simulink model "AdaptiveControlBuilding"  (R2017a)
settings: Solver=FixedStepAuto  StartTime=0  StopTime=75  MaxStep=0.5*Ts  RelTol=1e-3
values from neighbouring files (symbols this model uses):
  Ts = 1    [AdaptiveInitBuilding.m]    (also in Successive_Linearizer_Building.m = 0.5)
  u0 = [op_report.Inputs(1).u;op_report.Inputs(2).u]    [AdaptiveInitBuilding.m]
undefined symbols (not defined in the file or in its folder): K1, K10, K11, K12, K13, K14, K15, K2, K3, K4, K5, K6, K7, K8, K9
libraries: mpclib x1
settings Model: Creator=The MathWorks, Inc.  LastModifiedBy=gaobo1
settings DataIOCC: ExternalInput=ExtIn  InitialState=[311.267; 8.5695]  SaveFormat=Structure  SaveOutput=off  SignalLogging=off  SaveTime=off  SignalLoggingName=logsOut
settings OptimizationCC: BooleanDataType=off  DefaultParameterBehavior=Inlined  InlineInvariantSignals=on  BufferReuse=off  ExpressionDepthLimit=2147483647  InitFltsAndDblsToZero=on  LifeSpan=inf
settings DebuggingCC: SaveWithParameterizedLinksMsg=none  UnderspecifiedInitializationDetection=Classic  MergeDetectMultiDrivingBlocksExec=none  CheckExecutionContextPreStartOutputMsg=on  CheckExecutionContextRuntimeOutputMsg=on  SignalResolutionControl=TryResolveAllWithWarning  MultiTaskDSMMsg=warning  MultiTaskCondExecSysMsg=none  StateNameClashWarn=warning  SFUnexpectedBacktrackingDiag=warning  SFNoUnconditionalDefaultTransitionDiag=warning  SFExecutionAtInitializationDiag=none
settings HardwareCC: ProdBitPerPointer=32  ProdBitPerSizeT=32  ProdBitPerPtrDiffT=32  ProdLargestAtomicFloat=None  ProdIntDivRoundTo=Undefined  ProdEndianess=Unspecified  ProdWordSize=32  ProdHWDeviceType=32-bit Generic  TargetBitPerLong=64  TargetBitPerPointer=64  TargetBitPerSizeT=64  TargetBitPerPtrDiffT=64  TargetLongLongMode=on  TargetIntDivRoundTo=Zero  TargetEndianess=LittleEndian  TargetWordSize=64  TargetHWDeviceType=MATLAB Host  ProdEqTarget=off
settings ModelReferenceCC: PropagateSignalLabelsOutOfModel=off
settings GRTTargetCC: TargetFcnLib=ansi_tfl_tmw.mat  TargetLangStandard=C89/C90 (ANSI)  GeneratePreprocessorConditionals=Disable all  CombineOutputUpdateFcns=off  GRTInterface=on
settings ConfigComp: CovMetricSettings=dw  CovHtmlReporting=on  CovSaveCumulativeToWorkspaceVar=on  CovSaveSingleToWorkspaceVar=on  CovExternalEMLEnable=off  CovSFcnEnable=off

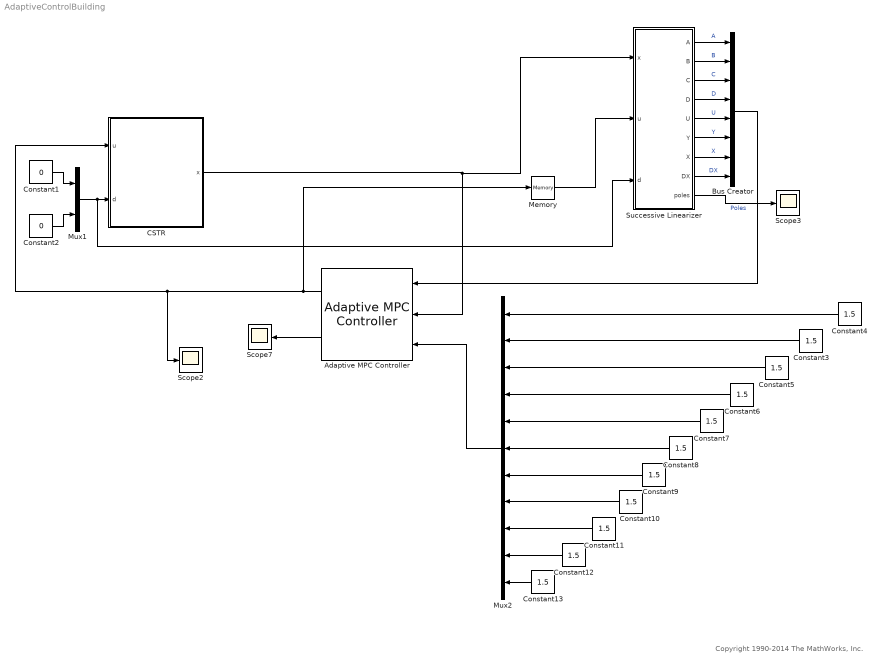
== system AdaptiveControlBuilding ==
  note: Copyright 1990-2014 The MathWorks, Inc.
  Adaptive MPC Controller : mpclib/Adaptive MPC Controller  SCDEnableBlockLinearizationSpecification=on  mpcobj=mpcobj  md_inport=off  mv_inport=off  cost_outport=off  return_sequence=off  return_qpstatus=off  return_state=on  state_inport=off  isltv_plant=off  lims_inport=off  ywt_inport=off  uwt_inport=off  duwt_inport=off  rhoeps_inport=off  uref_inport=off  BlockDataType=double  SampleTimeInherited=off  switch_inport=off
      settings: SourceProductName=Model Predictive Control Toolbox
  Bus Creator : BusCreator  Inputs=8
  CSTR : Subsystem
  Constant1 : Constant  Value=0
  Constant{3..13} (11 alike) : Constant  Value=1.5
  Constant2 : Constant  Value=0
  Memory : Memory  X0=u0
  Mux1 : Mux  Inputs=2
  Mux2 : Mux  Inputs=11
  Scope2 : Scope
  Scope3 : Scope
  Scope7 : Scope
  Successive Linearizer : MATLAB Function  TreatAsAtomicUnit=on  SystemSampleTime=Ts
  wires:
  Bus Creator/1 -> Adaptive MPC Controller/1
  Adaptive MPC Controller/1 -> Memory/1, CSTR/1(u), Scope2/1
  Successive Linearizer/1(A) -> Bus Creator/1  "A"
  Successive Linearizer/2(B) -> Bus Creator/2  "B"
  Successive Linearizer/3(C) -> Bus Creator/3  "C"
  Successive Linearizer/4(D) -> Bus Creator/4  "D"
  Successive Linearizer/5(U) -> Bus Creator/5  "U"
  Successive Linearizer/6(Y) -> Bus Creator/6  "Y"
  Successive Linearizer/7(X) -> Bus Creator/7  "X"
  Successive Linearizer/8(DX) -> Bus Creator/8  "DX"
  CSTR/1(x) -> Successive Linearizer/1(x), Adaptive MPC Controller/2
  Successive Linearizer/9(poles) -> Scope3/1  "Poles"
  Adaptive MPC Controller/2 -> Scope7/1
  Memory/1 -> Successive Linearizer/2(u)
  Constant1/1 -> Mux1/1
  Constant2/1 -> Mux1/2
  Mux1/1 -> Successive Linearizer/3(d), CSTR/2(d)
  Mux2/1 -> Adaptive MPC Controller/3
  Constant13/1 -> Mux2/11
  Constant12/1 -> Mux2/10
  Constant11/1 -> Mux2/9
  Constant10/1 -> Mux2/8
  Constant9/1 -> Mux2/7
  Constant8/1 -> Mux2/6
  Constant7/1 -> Mux2/5
  Constant6/1 -> Mux2/4
  Constant5/1 -> Mux2/3
  Constant3/1 -> Mux2/2
  Constant4/1 -> Mux2/1

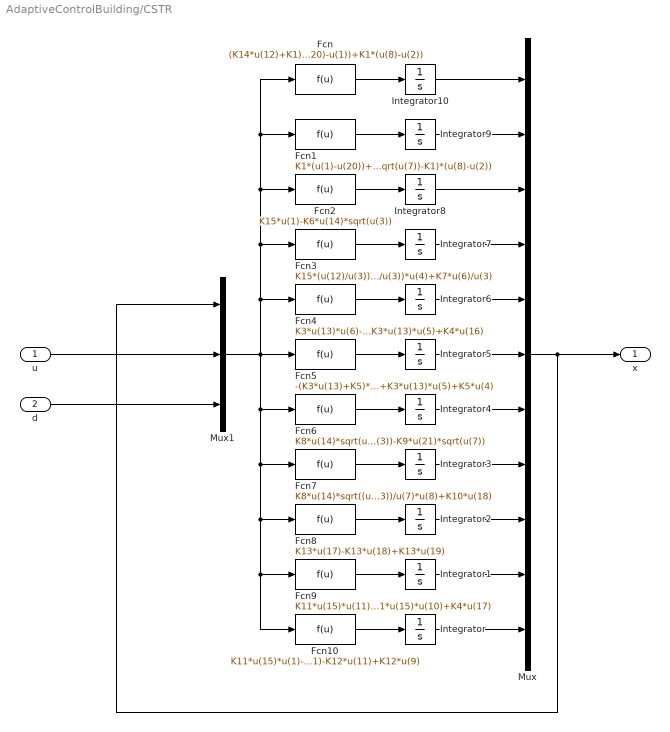
== system AdaptiveControlBuilding/CSTR ==
  u : Inport
  d : Inport  Port=2
  Fcn : Fcn  Expr=(K14*u(12)+K1)*(u(20)-u(1))+K1*(u(8)-u(2))
  Fcn1 : Fcn  Expr=K1*(u(1)-u(20))+(K2*u(21)*sqrt(u(7))-K1)*(u(8)-u(2))
  Fcn10 : Fcn  Expr=K11*u(15)*u(1)-K11*u(15)*u(11)-K12*u(11)+K12*u(9)
  Fcn2 : Fcn  Expr=K15*u(1)-K6*u(14)*sqrt(u(3))
  Fcn3 : Fcn  Expr=K15*(u(12)/u(3))*u(1)-(K15*(u(12)/u(3))+K7/u(3))*u(4)+K7*u(6)/u(3)
  Fcn4 : Fcn  Expr=K3*u(13)*u(6)-K3*u(13)*u(5)+K4*u(16)
  Fcn5 : Fcn  Expr=-(K3*u(13)+K5)*u(6)+K3*u(13)*u(5)+K5*u(4)
  Fcn6 : Fcn  Expr=K8*u(14)*sqrt(u(3))-K9*u(21)*sqrt(u(7))
  Fcn7 : Fcn  Expr=K8*u(14)*sqrt((u(3))/u(7)*u(4)-K8*u(14)*sqrt(u(3))/u(7)*u(8)+K10*u(18)
  Fcn8 : Fcn  Expr=K13*u(17)-K13*u(18)+K13*u(19)
  Fcn9 : Fcn  Expr=K11*u(15)*u(11)-K11*u(15)*u(10)+K4*u(17)
  Integrator{,1..10} (11 alike) : Integrator
  Mux : Mux  Inputs=11
  Mux1 : Mux  Inputs=3
  x : Outport
  wires:
  Integrator7/1 -> Mux/4
  Fcn2/1 -> Integrator8/1
  Fcn7/1 -> Integrator3/1
  Fcn/1 -> Integrator10/1
  Fcn6/1 -> Integrator4/1
  Integrator/1 -> Mux/11
  Fcn8/1 -> Integrator2/1
  Mux1/1 -> Fcn3/1, Fcn2/1, Fcn1/1, Fcn/1, Fcn4/1, Fcn5/1, Fcn6/1, Fcn8/1, Fcn10/1, Fcn9/1, Fcn7/1
  Mux/1 -> Mux1/1, x/1
  Integrator5/1 -> Mux/6
  Fcn3/1 -> Integrator7/1
  Integrator10/1 -> Mux/1
  Fcn9/1 -> Integrator1/1
  Integrator3/1 -> Mux/8
  d/1 -> Mux1/3
  Fcn5/1 -> Integrator5/1
  Integrator2/1 -> Mux/9
  u/1 -> Mux1/2
  Integrator1/1 -> Mux/10
  Fcn10/1 -> Integrator/1
  Integrator6/1 -> Mux/5
  Integrator8/1 -> Mux/3
  Integrator4/1 -> Mux/7
  Fcn1/1 -> Integrator9/1
  Fcn4/1 -> Integrator6/1
  Integrator9/1 -> Mux/2

== matlab function AdaptiveControlBuilding/Successive Linearizer ==
  data: A output size=[2,2]; x input; B output size=[2,2]; u input; d input; C output size=[2,2]; D output size=[2,2]; U output size=[2,1]; Y output size=[2,1]; X output size=[2,1]; DX output size=[2,1]; poles output size=[2 1]
% function [A, B, C, D, U, Y, X, DX, poles] = fcn(x1, x2, u1, u2)
% %#codegen
% 
% % Define constant outputs
% C = eye(2);
% D = zeros(2,2);
% % Nominal U are obtained from measurements
% U = [u1; u2];
% % Nominal X and Y are obtained from estimated MPC states
% Y = [x1; x2];
% X = [x1; x2];
% % Analytical linearization of mechanistic CSTR model (continuous time)
% 
% %%%%%%%%%%%%%%%%%%%%%%%%%%%%%%%%%%%%%%%%%%%%%%%%%%%%%%%%%%%%%%%%%%%%%%%%%
% %                   Initialization of State Vectors
% %%%%%%%%%%%%%%%%%%%%%%%%%%%%%%%%%%%%%%%%%%%%%%%%%%%%%%%%%%%%%%%%%%%%%%%%%
% n = 2;
% %%%%% Initial Conditions %%%%%
% % X0 = zeros(n,1);          % Equilibrium State X0 = [x10, x20, x30, ...]^T
% % X0(1) = 1.0;              % Initial Tank Level [m]
% % X0(2) = 81.5;             % Initial Tank Temperature (degC)
% % U0 = zeros(m,1);
% 
% %%%%% Definition of Constants %%%%%
% g = 9.81;           % Gravitational constant [m s^-2]
% T_C = 10;           % Cold water inlet temperature [degC]
% T_H = 90;           % Hot water inlet temperature [degC]
% A_o = 0.05;         % Outlet tank diameter [m^2]
% A_T = 3;            % Tank area [m^2]
% c_D = 0.7;          % Flow factor
% 
% %%%%%%%%%%%%%%%%%%%%%%%%%%%%%%%%%%%%%%%%%%%%%%%%%%%%%%%%%%%%%%%%%%%%%%%%%
% %                Linearization of the Nonlinear Tank System
% %%%%%%%%%%%%%%%%%%%%%%%%%%%%%%%%%%%%%%%%%%%%%%%%%%%%%%%%%%%%%%%%%%%%%%%%%
% Ue1 = c_D * A_o * sqrt(2*g*X(1)) * (T_H-X(2))/(T_H-T_C);   % Inlet cold water equi. flowrate        
% Ue2 = c_D * A_o * sqrt(2*g*X(1)) * (X(2)-T_C)/(T_H-T_C); 
% 
% Acts = [-c_D*A_o*sqrt(2*g/X(1))/(2*A_T) 0;
%     -(1/(A_T*X(1)^2))*(Ue1*(T_C-X(2))+Ue2*(T_H-X(2))) (1/(A_T*X(1)))*(-Ue1-Ue2)];
% 
% Bcts = [1/A_T 1/A_T;
%     (T_C-X(2))/(A_T*X(1)) (T_H-X(2))/(A_T*X(1)) ];
% 
% 
% %%%%%%%%%%%%%%%%%%%%%%%%%%%%%%%%%%%%%%%%%%%%%%%%%%%%%%%%%%%%%%%%%%%%%%%%%
% %               Discretization of the Continuous Time System
% %%%%%%%%%%%%%%%%%%%%%%%%%%%%%%%%%%%%%%%%%%%%%%%%%%%%%%%%%%%%%%%%%%%%%%%%%
% 
% % convert to discrete-time system
% Ts = 1;                                     % Sampling time
% Adis = expm(Ts*Acts);                       % Discretization of A matrix
% Bdis = (Acts\(expm(Ts*Acts)-eye(n)))*Bcts;  % Discretization of B matrix
% 
% % Last column of B contains the constant offset contribution.
% %DX = Bdis(:,3); 
% DX = [1/A_T*(Ue1+Ue2-c_D*A_o*sqrt(2*g*X(1))); 1/(A_T*X(1))*(Ue1*[T_C-X(2)]+Ue2*[T_H-X(2)])];
% 
% B = Bdis(:,1:2);
% A = Adis;
% % Compute poles
% poles = abs(eig(A));
% 
% end
function [A, B, C, D, U, Y, X, DX, poles] = fcn(x, u, d)
%#codegen

% Define constant outputs
Ts = 0.5;
C = eye(2);
D = zeros(2,2);
% Nominal U are obtained from measurements
U = [u1; u2];
% Nominal X and Y are obtained from estimated MPC states
Y = x;
X = y;
% Analytical linearization of mechanistic CSTR model (continuous time)
[A, Bo] = getContinuous(x, u, d);
% Convert continuous to discrete time
[A, Bo] = getDiscrete(A, Bo, Ts);
% Last column of B contains the constant offset contribution.
DX = Bo(:,3);
B = Bo(:,1:2);
% Compute poles
poles = abs(eig(A));

function [a, b] = getContinuous(X, U, Dist)
% Define linear continuous-time matrices A and B for CSTR.  Last input is
% offset.
K = zeros(15,1);
% Define constants
% Overall Model Constantsg = 9.81 * 1e2 * 3600^2;           % Gravitational constant [cm h^-2]
g = 9.81 * 1e2 * 3600^2;           % Gravitational constant [cm h^-2]
K_valve = 0.865;    % Valve coefficient conversion constant [to SI units]

rho_water = 1000 * 1e-6;   % Density of water [kg cm^-3]
rho_oil = 800 * 1e-6;      % Density of heating oil [kg cm^-3]
Cp_water = 4180 / 3600;    % Specific heat capacity of water [Wh kg^-1 K^-1]
Cp_oil = 1700 / 3600;      % Specific heat capacity of heating oil [Wh kg^-1 K^-1]

% Drain Water Heat Recovery (DWHR) Constants
n = 30;             % Number of internal tubes
d_tube = 0.01 * 1e2;      % Internal tube diameter [cm]
D_tube = 0.15 * 1e2;      % External tube diameter [cm]
L = 5 * 1e2;              % Tube(s) length [cm]
A_s_dwhr = n * pi * d_tube * L;              % Total surface area of internal tubes
V_dwhr_int = 0.25 * n * pi * L * d_tube^2;   % Total volume of internal tubes [m^3]
V_dwhr_tot = 0.25 * pi * L * D_tube^2;       % Volume of external tube [m^3]
V_dwhr_ext = V_dwhr_tot - V_dwhr_int;   % Volume of external tubes sans internal tubes [m^3]
V_dwhr_cold = V_dwhr_int;              % Cold water within internal tubes (for maintainability)
V_dwhr_hot = V_dwhr_ext;               % Hot water in external tube
U_dwhr = 1275 * 1e-4;                          % Overall heat transfer coefficient [W cm^-2 K^-1]

% Preheat Tank (PHT) Constants
H_pht_0 = 0.3 * 1e2;      % Initial level of PHT [cm]
H_pht_max = 1 * 1e2;      % Max height of PHT [cm]
A_pht = 0.01 * 1e4;       % Area of PHT [cm^2]
A_s_pht = 0.001 * 1e4;    % TODO Surface area of heating tube in PHT [cm^2]
U_pht = 1275 * 1e-4;       % TODO Overall heat transfer coefficient (PHT-LBTC) [W cm^-2 K^-1]
C_v_pht = 0.0167;   % Outlet valve coefficient

K(1) = U_dwhr * A_s_dwhr / (2 * rho_water * V_dwhr_cold * Cp_water); % [s^-1]
K(2) = K_valve * C_v_dhw * lambda / V_dwhr_hot; % [m^(-1/2) s^-1]
K(3) = Q_oil_tc / V_tube_tc; %[s^-1]
K(4) = 1 / (rho_oil * V_tube_tc * Cp_oil); % [J^-1 K]
K(5) = U_pht * A_s_pht / (rho_oil * V_tube_tc * Cp_oil); % [s^-1]
K(6) = K_valve * C_v_pht * lambda / A_pht; % [m^(-1/2) s^-1]
K(7) = U_pht * A_s_pht / (rho_water * Cp_water * A_pht); % [m s^-1]
K(8) = K_valve * C_v_pht * lambda / A_dhw; % [m^(-1/2) s^-1]
K(9) = K_valve * C_v_dhw * lambda / A_dhw; % [m^(-1/2) s^-1]
K(10) = 1 / (A_dhw * rho_water * Cp_water); % [J^-1 m K]
K(11) = Q_oil_tst / V_tube_tst; %[s^-1]
K(12) = U_tst * A_s_tst / (rho_water * V_tube_tst * Cp_oil); % [s^-1]
K(13) = 1 / (rho_water * Cp_water * V_tst); % [J^-1 K]
K(14) = 1 / V_dwhr_cold; % [m^-3]
K(15) = 1 / A_pht; % [m^-2]

% Nonlinear model time derivatives
dxdt = [(K(14)*U(1)+K(1))*Dist(1) - (K(14)*U(1)+K(1))*X(1)+ K(1)*X(8)-K(1)*X(2);
     -K(1)*Dist(1)+K(1)*X(1) + (K(2)*Dist(2)*sqrt(X(7)) - K(1))*X(8) - (K(2)*Dist(2)*sqrt(X(7)) - K(1))*X(2);
     K(15)*U(1) - K(6)*U(3)*sqrt(X(3));
     K(15)*U(1)*X(1)/X(3) - (K(15)*U(1)/X(3) + K(7)/X(3))*X(4) + K(7)*X(6)/X(3);
     K(3)*U(2)*X(6) - K(3)*U(2)*X(5) + K(4)*U(5);
     -(K(3)*U(2) + K(5))*X(6) + K(3)*U(2)*X(5) + K(5)*U(4);
     K(8)*U(3)*sqrt(X(3)) - K(9)*Dist(2)*sqrt(X(7));
     K(8)*U(3)*sqrt(X(3))*X(4)/X(7)-K(8)*U(3)*sqrt(X(3))*X(8)/X(7) + K(10)*U(7)/X(7);
     K(13)*U(6) - K(13)*U(7) + K(13) * U(8);
     K(11)*U(4)*X(11) - K(11)*U(4)*X(10) + K(4)*U(6);
     K(11)*U(4)*X(10) - (K(11)*U(4) + K(12))*X(11) + K(12)*X(9)];

a = [-K(1)-K(14)*U(1) -K(1) 0 0 0 0 0 K(1) 0 0 0;
    K(1) K(1)-Dist(2)*K(2)*sqrt(X(7)) 0 0 0 0 (Dist(2)*K(2)*X(8))/(2*sqrt(X(7)))-(Dist(2)*K(2)*X(2))/(2*sqrt(X(7))) Dist(2)*K2()*sqrt(X(7))-K(1) 0 0 0;
    0 0 -(K(6)*U(3))/(2*sqrt(X(3))) 0 0 0 0 0 0 0 0;
    K(15)*U(1)/X(3) 0 (X(4)*(K(7)+K(15)*U(1))-K(7)*X(6)-K(15)*U(1)*X(1))/(X(3)^2) -K(7)/X(3)-K(15)*U(1)/X(3) 0 K(7)/X(3) 0 0 0 0 0;
    0 0 0 0 -K(3)*U(2) K(3)*U(2) 0 0 0 0 0;
    0 0 0 0 K(3)*U(2) -K(5)-K(3)*U(2) 0 0 0 0 0;
    0 0 K(8)*U(3)/(2*sqrt(X(3))) 0 0 0 -Dist(2)*K(9)/(2*sqrt(X(7))) 0 0 0 0;
    0 0 (K(8)*U(3)*(X(4)-X(8)))/(2*sqrt(X(3))*X(7)) K(8)*U(3)*sqrt(X(3))/X(7) 0 0 K(8)*U(3)*sqrt(X(3))*(X(8)-X(4))/(X(7)^2) -K(8)*U(3)*sqrt(X(3))/X(7) 0 0 0;
    0 0 0 0 0 0 0 0 0 0 0;
    0 0 0 0 0 0 0 0 0 -K(11)*U(4) K(11)*U(4);
    0 0 0 0 0 0 0 0 K(12) K(11)*U(4) -K(12)-K11)*U(4)];

b = [Dist(1)*K(12)-K(12)*X(1) 0 0 0 0 0 0 0;
    0 0 0 0 0 0 0 0;
    K(15) 0 -K(6)*sqrt(X(3)) 0 0 0 0 0;
    K(15)*(X(1)-X(4))/X(3) 0 0 0 0 0 0 0;
    0 K(3)*X(6)-K(3)*X(5) 0 0 K(4) 0 0 0;
    0 K(3)*X(5)-K(3)*X(6) 0 K(5) 0 0 0 0;
    0 0 K(8)*sqrt(X(3)) 0 0 0 0 0;
    0 0 K(8)*sqrt(X(3))*(X(4)-X(8))/X(7) 0 0 0 K(10) 0;
    0 0 0 0 0 K(13) -K(13) K(13);
    0 0 0 K(11)*(X(11)-X(10)) 0 K(4) 0 0;
    0 0 0 K(11)*(X(10)-X(11)) 0 0 0 0];

b = [b dxdt];

% Make state indices consistent with x1 = h, x2 = T_T
% ix = [2,1];
% 
% a = a(ix,ix);
% b = b(ix,:);

function [A, B] = getDiscrete(a, b, Ts)
% Convert to discrete time
A = expm(a*Ts);
nx = size(b,1);
n = 4;  % Number of points for Simpson's Rule, an even integer >= 2.
% Use Simpson's rule to compute integral(0,Ts){expm(a*s)*ds*b}
h = Ts/n;
Ai = eye(nx) + A;        % First and last terms;
Coef = 2;
for i = 1:n-1
    if Coef == 2
        Coef = 4;
    else
        Coef = 2;
    end
    Ai = Ai + Coef*expm(a*i*h);     % Intermediate terms
end
B = (h/3)*Ai*b;
